simulink model "pendulum_model"  (R2019b)
settings: Solver=VariableStepAuto  StartTime=0.0  StopTime=30  MaxStep=0.015  RelTol=1e-3
values from neighbouring files (symbols this model uses):
  g = 10    [pendulum_workspace.mat]
  l = 1    [pendulum_workspace.mat]
  m = 20*log10([MinFreq MaxFreq])*Terms(i).multiplicity    [BodePlotGui.m]    (also in pendulum_workspace.mat = 100)
settings Model: Creator=Já  LastModifiedBy=Já

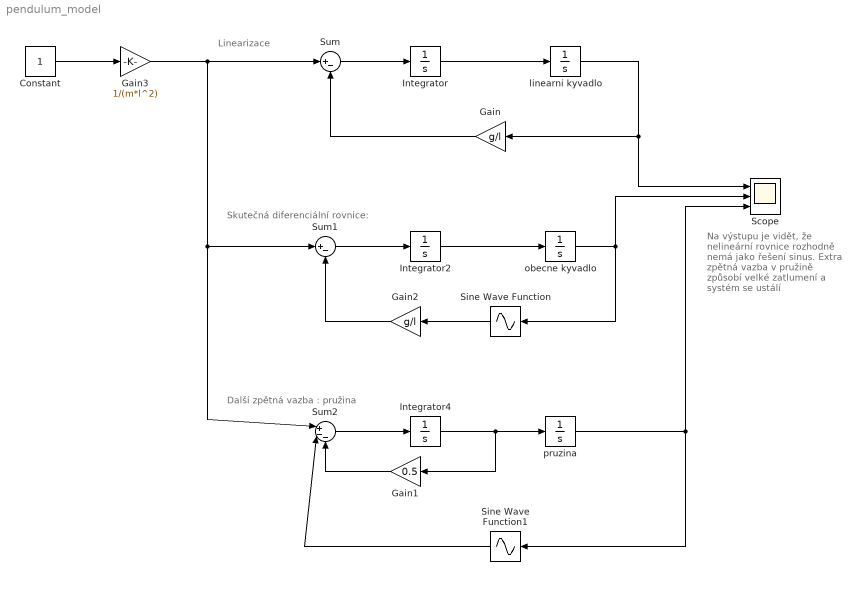
== system pendulum_model ==
  note: Na výstupu je vidět,
      | že nelineární rovnice
      | rozhodně nemá jako
      | řešení sinus.
      |
      | Extra zpětná vazba
      | v pružině způsobí velké
      | zatlumení a systém se ustálí
  note: Linearizace
  note: Skutečná diferenciální rovnice:
  note: Další zpětná vazba : pružina
  Constant : Constant
  Gain : Gain  Gain=g/l
  Gain1 : Gain  Gain=0.5
  Gain2 : Gain  Gain=g/l
  Gain3 : Gain  Gain=1/(m*l^2)
  Integrator : Integrator
  Integrator2 : Integrator
  Integrator4 : Integrator
  Scope : Scope  NumInputPorts=3
  Sine Wave Function : Sin  TimeSource=Use external signal  SampleTime=0
  Sine Wave Function1 : Sin  TimeSource=Use external signal  SampleTime=0
  Sum : Sum  Inputs=|+-
  Sum1 : Sum  Inputs=|+-
  Sum2 : Sum  Inputs=|+--
  linearni kyvadlo : Integrator  InitialCondition=3
  obecne kyvadlo : Integrator  InitialCondition=3
  pruzina : Integrator  InitialCondition=3
  wires:
  Integrator/1 -> linearni kyvadlo/1
  linearni kyvadlo/1 -> Scope/1, Gain/1
  Gain/1 -> Sum/2
  Sum/1 -> Integrator/1
  Sum1/1 -> Integrator2/1
  obecne kyvadlo/1 -> Sine Wave Function/1, Scope/2
  Integrator2/1 -> obecne kyvadlo/1
  Sine Wave Function/1 -> Gain2/1
  Sum2/1 -> Integrator4/1
  Integrator4/1 -> Gain1/1, pruzina/1
  Constant/1 -> Gain3/1
  pruzina/1 -> Sine Wave Function1/1, Scope/3
  Sine Wave Function1/1 -> Sum2/2
  Gain1/1 -> Sum2/3
  Gain2/1 -> Sum1/2
  Gain3/1 -> Sum2/1, Sum1/1, Sum/1
